simulink model "SF052A_SnsrOffsCorrn"  (R2013b)
settings: Solver=FixedStepDiscrete  SolverMode=SingleTasking  StartTime=0.0  StopTime=1  FixedStep=0.002  RelTol=1e-3
undefined symbols (not defined in the file): SnsrOffsCorrnHwAgLrndOffsLim, SnsrOffsCorrnHwTqLrndOffsLim, SnsrOffsCorrnOffsEna, SnsrOffsCorrnVehYawRateLrndOffsLim
libraries: NxtrLim x6, simulink x2
settings Model: Creator=SumitG  LastModifiedBy=TZ5743
settings SolverCC: AutoInsertRateTranBlk=on  InsertRTBMode=Always
settings DataIOCC: LimitDataPoints=off  SaveFormat=Structure  ReturnWorkspaceOutputs=on
settings OptimizationCC: BlockReduction=off  InlineParams=on  ZeroExternalMemoryAtStartup=off  ZeroInternalMemoryAtStartup=off  OptimizeModelRefInitCode=on  LifeSpan=1
settings DebuggingCC: SignalInfNanChecking=error  SignalRangeChecking=warning  UnderspecifiedInitializationDetection=Simplified  SolverPrmCheckMsg=error  InheritedTsInSrcMsg=error  DiscreteInheritContinuousMsg=error  SingleTaskRateTransMsg=error  TasksWithSamePriorityMsg=error  SigSpecEnsureSampleTimeMsg=error  CheckMatrixSingularityMsg=error  ParameterUnderflowMsg=error  ParameterPrecisionLossMsg=error  ParameterTunabilityLossMsg=error  FixptConstUnderflowMsg=warning  FixptConstOverflowMsg=warning  VectorMatrixConversionMsg=error  SignalLabelMismatchMsg=error  UnconnectedInputMsg=error  UnconnectedOutputMsg=error  UnconnectedLineMsg=error  SFcnCompatibilityMsg=error  UniqueDataStoreMsg=warning  BusObjectLabelMismatch=error  RootOutportRequireBusObject=error  AssertControl=DisableAll  ModelReferenceIOMsg=error  ModelReferenceVersionMismatchMessage=warning  ModelReferenceIOMismatchMessage=error  ModelReferenceCSMismatchMessage=warning  ModelReferenceDataLoggingMessage=error  StateNameClashWarn=warning  StrictBusMsg=ErrorOnBusTreatedAsVector  NonBusSignalsTreatedAsBus=error  SFUnexpectedBacktrackingDiag=error  SFInvalidInputDataAccessInChartInitDiag=error  SFNoUnconditionalDefaultTransitionDiag=error  SFTransitionOutsideNaturalParentDiag=error  SFUnconditionalTransitionShadowingDiag=error  SFUndirectedBroadcastEventsDiag=error
settings ModelReferenceCC: ModelReferenceNumInstancesAllowed=Single
settings RTWCC: SystemTargetFile=autosar.tlc  GenCodeOnly=on  TemplateMakefile=ert_default_tmf  Description=AUTOSAR  GenerateReport=on  ProcessScript=autosar_make_rtw_hook  LaunchReport=on
settings CodeAppCC: GenerateComments=off  IgnoreCustomStorageClasses=off  CustomSymbolStrType=$N$R$M  CustomSymbolStrBlkIO=$N$M  SimulinkBlockComments=off
settings STFCustomTargetCC: ParMdlRefBuildCompliant=on  CompOptLevelCompliant=on  IncludeMdlTerminateFcn=off  CombineOutputUpdateFcns=on  SuppressErrorStatus=on  ERTFirstTimeCompliant=on  ERTCustomFileBanners=on  SupportNonFinite=off  SupportComplex=off  SupportContinuousTime=off  SupportNonInlinedSFcns=off  MATLABClassNameForMDSCustomization=Simulink.SoftwareTarget.ERTCustomization  AutosarCompliant=on  GRTInterface=off  SystemTargetFile=autosar.tlc
settings ERTTargetCC: CodeReplacementLibrary=ANSI_C  ConcurrentExecutionCompliant=off  IncludeMdlTerminateFcn=off  SuppressErrorStatus=on  SupportNonFinite=off  SupportComplex=off  ModelStepFunctionPrototypeControlCompliant=off  CPPClassGenCompliant=off  AutosarCompliant=on  InlinedParameterPlacement=NonHierarchical  ERTCustomFileTemplate=example_file_process.tlc  EnableUserReplacementTypes=on

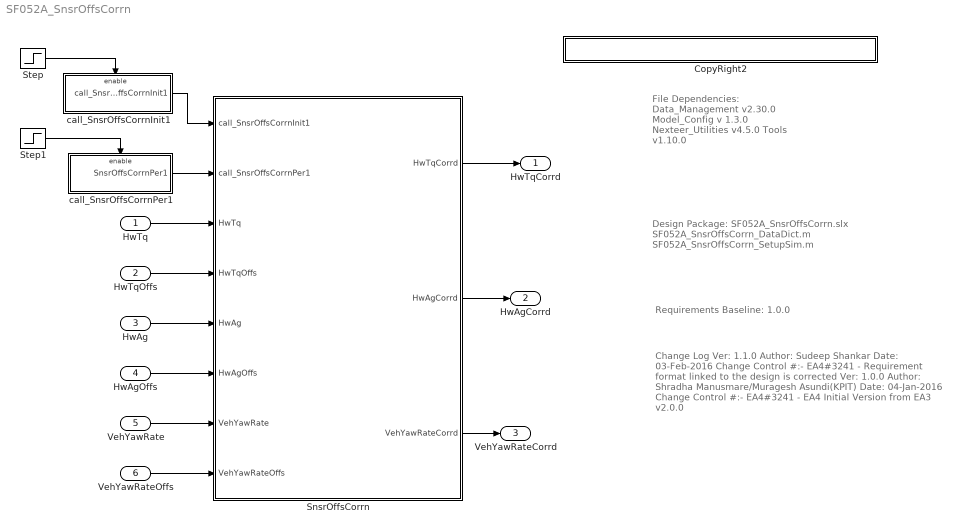
== system SF052A_SnsrOffsCorrn ==
  note: File Dependencies:
      |
      | Data_Management v2.30.0
      | Model_Config v 1.3.0
      | Nexteer_Utilities v4.5.0
      | Tools v1.10.0
  note: Requirements Baseline: 1.0.0
  note: Design Package:
      | SF052A_SnsrOffsCorrn.slx
      | SF052A_SnsrOffsCorrn_DataDict.m
      | SF052A_SnsrOffsCorrn_SetupSim.m
  note: Change Log
      |
      | Ver: 1.1.0
      | Author: Sudeep Shankar
      | Date: 03-Feb-2016
      | Change Control #:- EA4#3241
      | - Requirement format linked to the design is corrected
      |
      | Ver: 1.0.0
      | Author: Shradha Manusmare/Muragesh Asundi(KPIT)
      | Date: 04-Jan-2016
      | Change Control #:- EA4#3241
      | - EA4 Initial Version from EA3 v2.0.0
  HwTq : Inport  RequirementInfo={} %GIDa_2cd6e272_0df7_4175_9761_7c22e4c47b1c
  HwTqOffs : Inport  RequirementInfo={} %GIDa_54a2ce7e_9bb3_43b4_b9bf_3347b6fc5bcb  Port=2
  HwAg : Inport  RequirementInfo={} %GIDa_eed449fb_96e4_4476_834f_f50e1c62bf51  Port=3
  HwAgOffs : Inport  RequirementInfo={} %GIDa_50720404_89e5_4c59_9f63_6b50f8eae543  Port=4
  VehYawRate : Inport  RequirementInfo={} %GIDa_c6d0fb8d_2bf0_45a9_af32_27cacd4678ab  Port=5
  VehYawRateOffs : Inport  RequirementInfo={} %GIDa_e4fac660_fc81_4d67_abb0_5d2918f20bf2  Port=6
  CopyRight2 : Subsystem  Description=|  mask(Copyright Information){none=on}
      | Copyright info block.                                               
      |                                                                     
      | Place copyright information at the top of every subsystem in design.
      mask prompts: none "No parameters"
      mask help: Place copyright information at the top of every subsystem in design.
      mask Display:
      | NxtrConf = 'Nexteer Confidential';
      | 
      | sys = bdroot; %handle for the current model ("system")
      | first = get_param(sys,'Created');
      | first = first(end-3:end);  %year is last four digits
      | 
      | last = get_param(sys,'LastModifiedDate');
      | if isempty(last)
      |     last = datestr(now,'yyyy');
      | else
      |     last = last(end-3:end);
      | end
      | 
      | if strcmp(first,last)
      |     fprintf('%s -- Copyright %s Nexteer',NxtrConf,first)
      | else
      |     fprintf('%s -- %s%s- %s Nexteer',NxtrConf,char(169),first,last)
      | end
  SnsrOffsCorrn : Subsystem  RequirementInfo="{'linktype_rmi_doors' '0000bab4 (/E-STEER Core/SubSystem Specifications/Application Functions/SF052A Sensor Offset Correction  v0p2 150831)' '#SF052A_10' 'true' 'REQ:  SF052A_10' '' } %GIDa_ea5d6bfe_7895_439c_b9de_069ac848c9e6"
  Step : Step  Before=1  After=0  SampleTime=0
  Step1 : Step  SampleTime=0
  call_SnsrOffsCorrnInit1 : Subsystem  TreatAsAtomicUnit=on
  call_SnsrOffsCorrnPer1 : Subsystem  TreatAsAtomicUnit=on
  HwTqCorrd : Outport
  HwAgCorrd : Outport  Port=2
  VehYawRateCorrd : Outport  Port=3
  wires:
  SnsrOffsCorrn/3(VehYawRateCorrd) -> VehYawRateCorrd/1
  SnsrOffsCorrn/2(HwAgCorrd) -> HwAgCorrd/1
  SnsrOffsCorrn/1(HwTqCorrd) -> HwTqCorrd/1
  call_SnsrOffsCorrnInit1/1(call_SnsrOffsCorrnInit1) -> SnsrOffsCorrn/1(call_SnsrOffsCorrnInit1)
  HwAgOffs/1 -> SnsrOffsCorrn/6(HwAgOffs)
  VehYawRateOffs/1 -> SnsrOffsCorrn/8(VehYawRateOffs)
  VehYawRate/1 -> SnsrOffsCorrn/7(VehYawRate)
  HwAg/1 -> SnsrOffsCorrn/5(HwAg)
  HwTqOffs/1 -> SnsrOffsCorrn/4(HwTqOffs)
  HwTq/1 -> SnsrOffsCorrn/3(HwTq)
  Step/1 -> call_SnsrOffsCorrnInit1/Enable
  call_SnsrOffsCorrnPer1/1(SnsrOffsCorrnPer1) -> SnsrOffsCorrn/2(call_SnsrOffsCorrnPer1)
  Step1/1 -> call_SnsrOffsCorrnPer1/Enable

== system SF052A_SnsrOffsCorrn/CopyRight2 ==

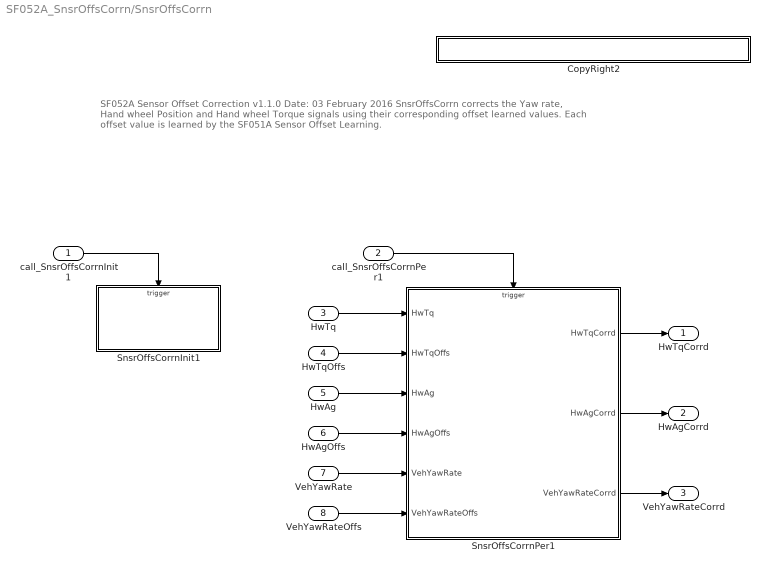
== system SF052A_SnsrOffsCorrn/SnsrOffsCorrn ==
  note: SF052A  Sensor Offset Correction
      | v1.1.0 								                                                                     Date: 03 February 2016
      |
      | SnsrOffsCorrn corrects the Yaw rate, Hand wheel Position and Hand wheel Torque signals using their
      | corresponding offset learned values. Each offset value is learned by the SF051A Sensor Offset Learning.
  call_SnsrOffsCorrnInit1 : Inport
  call_SnsrOffsCorrnPer1 : Inport  RequirementInfo="{'linktype_rmi_doors' '0000bab4 (/E-STEER Core/SubSystem Specifications/Application Functions/SF052A Sensor Offset Correction  v0p2 150831)' '#SF052A_56' 'true' 'REQ:  SF052A_56' '' } %GIDa_c7ebcd4c_7a0e_430e_914f_69a33bdc4f8e"  Port=2
  HwTq : Inport  RequirementInfo="{'linktype_rmi_doors' '0000bab4 (/E-STEER Core/SubSystem Specifications/Application Functions/SF052A Sensor Offset Correction  v0p2 150831)' '#SF052A_10' 'true' 'REQ:  SF052A_10' '' } %GIDa_886c7520_3b64_4a4e_b91f_bd52fc6cdafc"  Port=3
  HwTqOffs : Inport  RequirementInfo="{'linktype_rmi_doors' '0000bab4 (/E-STEER Core/SubSystem Specifications/Application Functions/SF052A Sensor Offset Correction  v0p2 150831)' '#SF052A_13' 'true' 'REQ:  SF052A_13' '' } %GIDa_0789263f_55f5_4e30_882e_ed1743b93406"  Port=4
  HwAg : Inport  RequirementInfo="{'linktype_rmi_doors' '0000bab4 (/E-STEER Core/SubSystem Specifications/Application Functions/SF052A Sensor Offset Correction  v0p2 150831)' '#SF052A_11' 'true' 'REQ:  SF052A_11' '' } %GIDa_98e8cd6b_ab1c_44ad_b544_e07a839ca543"  Port=5
  HwAgOffs : Inport  RequirementInfo="{'linktype_rmi_doors' '0000bab4 (/E-STEER Core/SubSystem Specifications/Application Functions/SF052A Sensor Offset Correction  v0p2 150831)' '#SF052A_14' 'true' 'REQ:  SF052A_14' '' } %GIDa_35d31cf1_93f6_46eb_aefe_bfa7895b93aa"  Port=6
  VehYawRate : Inport  RequirementInfo="{'linktype_rmi_doors' '0000bab4 (/E-STEER Core/SubSystem Specifications/Application Functions/SF052A Sensor Offset Correction  v0p2 150831)' '#SF052A_12' 'true' 'REQ:  SF052A_12' '' } %GIDa_f163533a_1fd4_4cf7_966b_304b3abdf020"  Port=7
  VehYawRateOffs : Inport  RequirementInfo="{'linktype_rmi_doors' '0000bab4 (/E-STEER Core/SubSystem Specifications/Application Functions/SF052A Sensor Offset Correction  v0p2 150831)' '#SF052A_15' 'true' 'REQ:  SF052A_15' '' } %GIDa_349c3e39_d0d8_4839_8edd_a04b0f97528a"  Port=8
  CopyRight2 : Subsystem  Description=|  mask(Copyright Information){none=on}
      | Copyright info block.                                               
      |                                                                     
      | Place copyright information at the top of every subsystem in design.
      mask prompts: none "No parameters"
      mask help: Place copyright information at the top of every subsystem in design.
      mask Display:
      | NxtrConf = 'Nexteer Confidential';
      | 
      | sys = bdroot; %handle for the current model ("system")
      | first = get_param(sys,'Created');
      | first = first(end-3:end);  %year is last four digits
      | 
      | last = get_param(sys,'LastModifiedDate');
      | if isempty(last)
      |     last = datestr(now,'yyyy');
      | else
      |     last = last(end-3:end);
      | end
      | 
      | if strcmp(first,last)
      |     fprintf('%s -- Copyright %s Nexteer',NxtrConf,first)
      | else
      |     fprintf('%s -- %s%s- %s Nexteer',NxtrConf,char(169),first,last)
      | end
  SnsrOffsCorrnInit1 : Subsystem  TreatAsAtomicUnit=on
  SnsrOffsCorrnPer1 : Subsystem  TreatAsAtomicUnit=on
  HwTqCorrd : Outport  RequirementInfo="{'linktype_rmi_doors' '0000bab4 (/E-STEER Core/SubSystem Specifications/Application Functions/SF052A Sensor Offset Correction  v0p2 150831)' '#SF052A_17' 'true' 'REQ:  SF052A_17' '' } %GIDa_182c97d9_5f7d_4d89_81b8_b7d4c7ce856d"
  HwAgCorrd : Outport  RequirementInfo="{'linktype_rmi_doors' '0000bab4 (/E-STEER Core/SubSystem Specifications/Application Functions/SF052A Sensor Offset Correction  v0p2 150831)' '#SF052A_18' 'true' 'REQ:  SF052A_18' '' } %GIDa_122c88ba_5244_46f5_838e_7cffdb4a64bf"  Port=2
  VehYawRateCorrd : Outport  RequirementInfo="{'linktype_rmi_doors' '0000bab4 (/E-STEER Core/SubSystem Specifications/Application Functions/SF052A Sensor Offset Correction  v0p2 150831)' '#SF052A_19' 'true' 'REQ:  SF052A_19' '' } %GIDa_98fd8efd_54d6_4bd4_9a2d_dfa8e7aa3144"  Port=3
  wires:
  call_SnsrOffsCorrnPer1/1 -> SnsrOffsCorrnPer1/Trigger
  SnsrOffsCorrnPer1/1(HwTqCorrd) -> HwTqCorrd/1
  SnsrOffsCorrnPer1/2(HwAgCorrd) -> HwAgCorrd/1
  SnsrOffsCorrnPer1/3(VehYawRateCorrd) -> VehYawRateCorrd/1
  VehYawRateOffs/1 -> SnsrOffsCorrnPer1/6(VehYawRateOffs)
  VehYawRate/1 -> SnsrOffsCorrnPer1/5(VehYawRate)
  HwAgOffs/1 -> SnsrOffsCorrnPer1/4(HwAgOffs)
  HwAg/1 -> SnsrOffsCorrnPer1/3(HwAg)
  HwTqOffs/1 -> SnsrOffsCorrnPer1/2(HwTqOffs)
  HwTq/1 -> SnsrOffsCorrnPer1/1(HwTq)
  call_SnsrOffsCorrnInit1/1 -> SnsrOffsCorrnInit1/Trigger

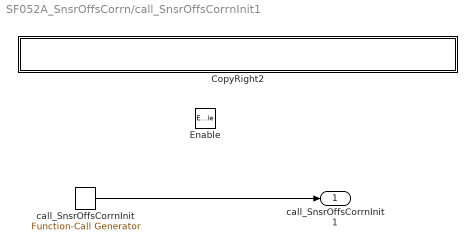
== system SF052A_SnsrOffsCorrn/call_SnsrOffsCorrnInit1 ==
  Enable : EnablePort
  CopyRight2 : Subsystem  Description=|  mask(Copyright Information){none=on}
      | Copyright info block.                                               
      |                                                                     
      | Place copyright information at the top of every subsystem in design.
      mask prompts: none "No parameters"
      mask help: Place copyright information at the top of every subsystem in design.
      mask Display:
      | NxtrConf = 'Nexteer Confidential';
      | 
      | sys = bdroot; %handle for the current model ("system")
      | first = get_param(sys,'Created');
      | first = first(end-3:end);  %year is last four digits
      | 
      | last = get_param(sys,'LastModifiedDate');
      | if isempty(last)
      |     last = datestr(now,'yyyy');
      | else
      |     last = last(end-3:end);
      | end
      | 
      | if strcmp(first,last)
      |     fprintf('%s -- Copyright %s Nexteer',NxtrConf,first)
      | else
      |     fprintf('%s -- %s%s- %s Nexteer',NxtrConf,char(169),first,last)
      | end
  "call_SnsrOffsCorrnInit " : simulink/Ports & Subsystems/Function-Call Generator  sample_time=0  numberOfIterations=1
  call_SnsrOffsCorrnInit1 : Outport
  wires:
  "call_SnsrOffsCorrnInit "/1 -> call_SnsrOffsCorrnInit1/1

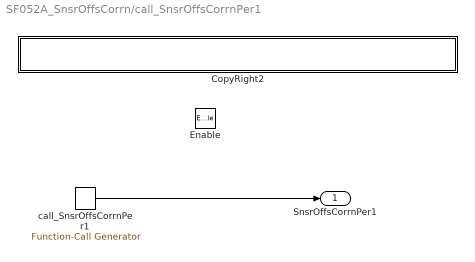
== system SF052A_SnsrOffsCorrn/call_SnsrOffsCorrnPer1 ==
  Enable : EnablePort
  CopyRight2 : Subsystem  Description=|  mask(Copyright Information){none=on}
      | Copyright info block.                                               
      |                                                                     
      | Place copyright information at the top of every subsystem in design.
      mask prompts: none "No parameters"
      mask help: Place copyright information at the top of every subsystem in design.
      mask Display:
      | NxtrConf = 'Nexteer Confidential';
      | 
      | sys = bdroot; %handle for the current model ("system")
      | first = get_param(sys,'Created');
      | first = first(end-3:end);  %year is last four digits
      | 
      | last = get_param(sys,'LastModifiedDate');
      | if isempty(last)
      |     last = datestr(now,'yyyy');
      | else
      |     last = last(end-3:end);
      | end
      | 
      | if strcmp(first,last)
      |     fprintf('%s -- Copyright %s Nexteer',NxtrConf,first)
      | else
      |     fprintf('%s -- %s%s- %s Nexteer',NxtrConf,char(169),first,last)
      | end
  "call_SnsrOffsCorrnPer1 " : simulink/Ports & Subsystems/Function-Call Generator  sample_time=0  numberOfIterations=1
  SnsrOffsCorrnPer1 : Outport
  wires:
  "call_SnsrOffsCorrnPer1 "/1 -> SnsrOffsCorrnPer1/1

== system SF052A_SnsrOffsCorrn/SnsrOffsCorrn/CopyRight2 ==

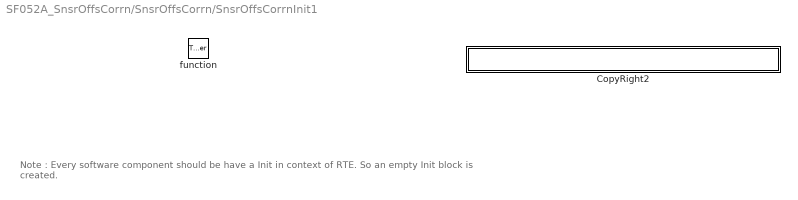
== system SF052A_SnsrOffsCorrn/SnsrOffsCorrn/SnsrOffsCorrnInit1 ==
  note: Note : Every software component should be have a Init in context of RTE. So an empty Init block is created.
  function : TriggerPort  TriggerType=function-call
  CopyRight2 : Subsystem  Description=|  mask(Copyright Information){none=on}
      | Copyright info block.                                               
      |                                                                     
      | Place copyright information at the top of every subsystem in design.
      mask prompts: none "No parameters"
      mask help: Place copyright information at the top of every subsystem in design.
      mask Display:
      | NxtrConf = 'Nexteer Confidential';
      | 
      | sys = bdroot; %handle for the current model ("system")
      | first = get_param(sys,'Created');
      | first = first(end-3:end);  %year is last four digits
      | 
      | last = get_param(sys,'LastModifiedDate');
      | if isempty(last)
      |     last = datestr(now,'yyyy');
      | else
      |     last = last(end-3:end);
      | end
      | 
      | if strcmp(first,last)
      |     fprintf('%s -- Copyright %s Nexteer',NxtrConf,first)
      | else
      |     fprintf('%s -- %s%s- %s Nexteer',NxtrConf,char(169),first,last)
      | end

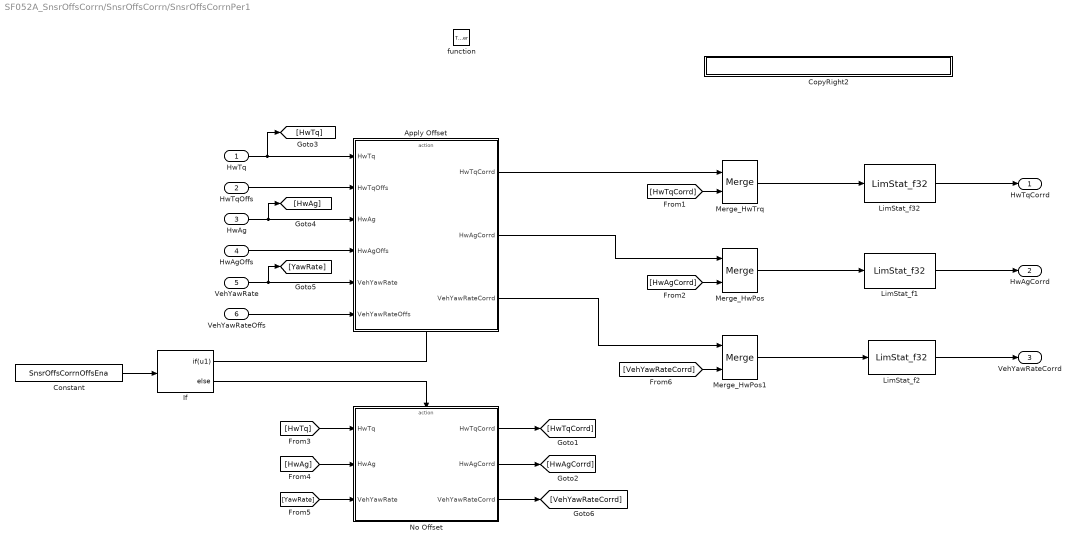
== system SF052A_SnsrOffsCorrn/SnsrOffsCorrn/SnsrOffsCorrnPer1 ==
  HwTq : Inport
  HwTqOffs : Inport  Port=2
  HwAg : Inport  Port=3
  HwAgOffs : Inport  Port=4
  VehYawRate : Inport  Port=5
  VehYawRateOffs : Inport  Port=6
  function : TriggerPort  TriggerType=function-call
  Apply Offset : Subsystem  TreatAsAtomicUnit=on
  Constant : Constant  RequirementInfo="{'linktype_rmi_doors' '0000bab4 (/E-STEER Core/SubSystem Specifications/Application Functions/SF052A Sensor Offset Correction  v0p2 150831)' '#SF052A_59' 'true' 'REQ:  SF052A_59' '' } %GIDa_2ea6c251_add8_4fde_8222_930c6875a31a"  Value=SnsrOffsCorrnOffsEna  OutDataTypeStr=boolean
  CopyRight2 : Subsystem  Description=|  mask(Copyright Information){none=on}
      | Copyright info block.                                               
      |                                                                     
      | Place copyright information at the top of every subsystem in design.
      mask prompts: none "No parameters"
      mask help: Place copyright information at the top of every subsystem in design.
      mask Display:
      | NxtrConf = 'Nexteer Confidential';
      | 
      | sys = bdroot; %handle for the current model ("system")
      | first = get_param(sys,'Created');
      | first = first(end-3:end);  %year is last four digits
      | 
      | last = get_param(sys,'LastModifiedDate');
      | if isempty(last)
      |     last = datestr(now,'yyyy');
      | else
      |     last = last(end-3:end);
      | end
      | 
      | if strcmp(first,last)
      |     fprintf('%s -- Copyright %s Nexteer',NxtrConf,first)
      | else
      |     fprintf('%s -- %s%s- %s Nexteer',NxtrConf,char(169),first,last)
      | end
  If : If  RequirementInfo="{'linktype_rmi_doors' '0000bab4 (/E-STEER Core/SubSystem Specifications/Application Functions/SF052A Sensor Offset Correction  v0p2 150831)' '#SF052A_59' 'true' 'REQ:  SF052A_59' '' } %GIDa_2324c2e3_bcd9_4140_a9db_9a8142331170"  IfExpression=u1
  LimStat_f1 : NxtrLim/LimStat_f32  RequirementInfo="{'linktype_rmi_doors' '0000bab4 (/E-STEER Core/SubSystem Specifications/Application Functions/SF052A Sensor Offset Correction  v0p2 150831)' '#SF052A_36' 'true' 'REQ:  SF052A_36' '' } %GIDa_c146a09b_42a0_4475_9c71_a8af706049e4"  LoLim=HWAGLOLIM_HWDEG_F32  HiLim=HWAGHILIM_HWDEG_F32
      settings: AttributesFormatString=|
      | Low Limit: %<LoLim>
      | High Limit:%<HiLim>
  LimStat_f2 : NxtrLim/LimStat_f32  RequirementInfo="{'linktype_rmi_doors' '0000bab4 (/E-STEER Core/SubSystem Specifications/Application Functions/SF052A Sensor Offset Correction  v0p2 150831)' '#SF052A_37' 'true' 'REQ:  SF052A_37' '' } %GIDa_c30e3b2b_2f7c_4b91_b252_a338ad55317b"  LoLim=VEHYAWRATELOLIM_VEHDEGPERSEC_F32  HiLim=VEHYAWRATEHILIM_VEHDEGPERSEC_F32
      settings: AttributesFormatString=|
      | Low Limit: %<LoLim>
      | High Limit:%<HiLim>
  LimStat_f32 : NxtrLim/LimStat_f32  RequirementInfo="{'linktype_rmi_doors' '0000bab4 (/E-STEER Core/SubSystem Specifications/Application Functions/SF052A Sensor Offset Correction  v0p2 150831)' '#SF052A_35' 'true' 'REQ:  SF052A_35' '' } %GIDa_66be3942_6c95_4b2c_b34d_b042724e9ab2"  LoLim=ELECGLBPRM_HWTQSATNLOWRLIM_HWNWTMTR_F32  HiLim=ELECGLBPRM_HWTQSATNUPPRLIM_HWNWTMTR_F32
      settings: AttributesFormatString=|
      | Low Limit: %<LoLim>
      | High Limit:%<HiLim>
  Merge_HwPos : Merge
  Merge_HwPos1 : Merge
  Merge_HwTrq : Merge
  No Offset : Subsystem  TreatAsAtomicUnit=on
  HwTqCorrd : Outport
  HwAgCorrd : Outport  Port=2
  VehYawRateCorrd : Outport  Port=3
  wires:
  Constant/1 -> If/1
  Merge_HwTrq/1 -> LimStat_f32/1
  LimStat_f32/1 -> HwTqCorrd/1
  Merge_HwPos/1 -> LimStat_f1/1
  LimStat_f1/1 -> HwAgCorrd/1
  Merge_HwPos1/1 -> LimStat_f2/1
  LimStat_f2/1 -> VehYawRateCorrd/1
  HwTq/1 -> [HwTq], Apply Offset/1(HwTq)
  HwTqOffs/1 -> Apply Offset/2(HwTqOffs)
  HwAg/1 -> Apply Offset/3(HwAg), [HwAg]
  HwAgOffs/1 -> Apply Offset/4(HwAgOffs)
  VehYawRate/1 -> [YawRate], Apply Offset/5(VehYawRate)
  VehYawRateOffs/1 -> Apply Offset/6(VehYawRateOffs)
  If/1 -> Apply Offset/Action
  [HwTq] -> No Offset/1(HwTq)
  [HwAg] -> No Offset/2(HwAg)
  [YawRate] -> No Offset/3(VehYawRate)
  If/2 -> No Offset/Action
  Apply Offset/1(HwTqCorrd) -> Merge_HwTrq/1
  Apply Offset/2(HwAgCorrd) -> Merge_HwPos/1
  Apply Offset/3(VehYawRateCorrd) -> Merge_HwPos1/1
  No Offset/1(HwTqCorrd) -> [HwTqCorrd]
  No Offset/2(HwAgCorrd) -> [HwAgCorrd]
  No Offset/3(VehYawRateCorrd) -> [VehYawRateCorrd]
  [HwTqCorrd] -> Merge_HwTrq/2
  [HwAgCorrd] -> Merge_HwPos/2
  [VehYawRateCorrd] -> Merge_HwPos1/2

== system SF052A_SnsrOffsCorrn/call_SnsrOffsCorrnInit1/CopyRight2 ==

== system SF052A_SnsrOffsCorrn/call_SnsrOffsCorrnPer1/CopyRight2 ==

== system SF052A_SnsrOffsCorrn/SnsrOffsCorrn/SnsrOffsCorrnInit1/CopyRight2 ==

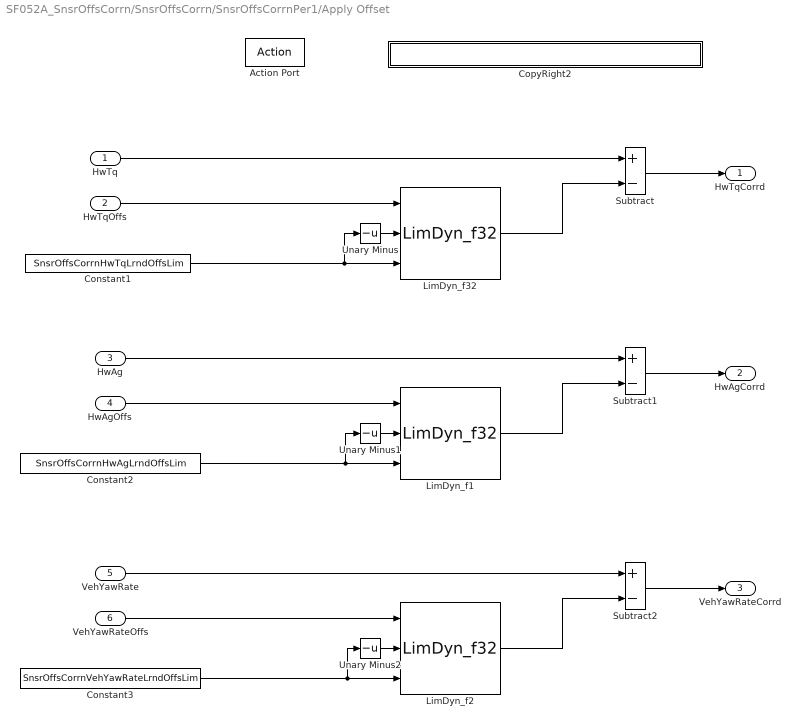
== system SF052A_SnsrOffsCorrn/SnsrOffsCorrn/SnsrOffsCorrnPer1/Apply Offset ==
  HwTq : Inport
  HwTqOffs : Inport  RequirementInfo={} %GIDa_208833cf_6878_470b_b6db_b869c72ce382  Port=2
  HwAg : Inport  Port=3
  HwAgOffs : Inport  RequirementInfo={} %GIDa_13fd176b_bd90_4d1e_898c_b4cb84dd90d3  Port=4
  VehYawRate : Inport  Port=5
  VehYawRateOffs : Inport  RequirementInfo={} %GIDa_c6aad98d_57dc_4e55_93b2_43b7f5e68072  Port=6
  Action Port : ActionPort  ActionType=then
  Constant1 : Constant  RequirementInfo="{'linktype_rmi_doors' '0000bab4 (/E-STEER Core/SubSystem Specifications/Application Functions/SF052A Sensor Offset Correction  v0p2 150831)' '#SF052A_28' 'true' 'REQ:  SF052A_28' '' ; 'linktype_rmi_doors' '0000bab4 (/E-STEER Core/SubSystem Specifications/Application Functions/SF052A Sensor Offset Correction  v0p2 150831)' '#SF052A_59' 'true' 'REQ:  SF052A_59' '' } %GIDa_c02cbdf8_d780_4ec2_988f_a7f581d45f4e"  Value=SnsrOffsCorrnHwTqLrndOffsLim  OutDataTypeStr=single
  Constant2 : Constant  RequirementInfo="{'linktype_rmi_doors' '0000bab4 (/E-STEER Core/SubSystem Specifications/Application Functions/SF052A Sensor Offset Correction  v0p2 150831)' '#SF052A_29' 'true' 'REQ:  SF052A_29' '' ; 'linktype_rmi_doors' '0000bab4 (/E-STEER Core/SubSystem Specifications/Application Functions/SF052A Sensor Offset Correction  v0p2 150831)' '#SF052A_59' 'true' 'REQ:  SF052A_59' '' } %GIDa_84e76d09_10c3_4f45_963b_f70ffbb4b24a"  Value=SnsrOffsCorrnHwAgLrndOffsLim  OutDataTypeStr=single
  Constant3 : Constant  RequirementInfo="{'linktype_rmi_doors' '0000bab4 (/E-STEER Core/SubSystem Specifications/Application Functions/SF052A Sensor Offset Correction  v0p2 150831)' '#SF052A_30' 'true' 'REQ:  SF052A_30' '' ; 'linktype_rmi_doors' '0000bab4 (/E-STEER Core/SubSystem Specifications/Application Functions/SF052A Sensor Offset Correction  v0p2 150831)' '#SF052A_59' 'true' 'REQ:  SF052A_59' '' } %GIDa_e3eda51d_9ed4_441b_9c35_48416a4bd64d"  Value=SnsrOffsCorrnVehYawRateLrndOffsLim  OutDataTypeStr=single
  CopyRight2 : Subsystem  Description=|  mask(Copyright Information){none=on}
      | Copyright info block.                                               
      |                                                                     
      | Place copyright information at the top of every subsystem in design.
      mask prompts: none "No parameters"
      mask help: Place copyright information at the top of every subsystem in design.
      mask Display:
      | NxtrConf = 'Nexteer Confidential';
      | 
      | sys = bdroot; %handle for the current model ("system")
      | first = get_param(sys,'Created');
      | first = first(end-3:end);  %year is last four digits
      | 
      | last = get_param(sys,'LastModifiedDate');
      | if isempty(last)
      |     last = datestr(now,'yyyy');
      | else
      |     last = last(end-3:end);
      | end
      | 
      | if strcmp(first,last)
      |     fprintf('%s -- Copyright %s Nexteer',NxtrConf,first)
      | else
      |     fprintf('%s -- %s%s- %s Nexteer',NxtrConf,char(169),first,last)
      | end
  LimDyn_f1 : NxtrLim/LimDyn_f32
  LimDyn_f2 : NxtrLim/LimDyn_f32
  LimDyn_f32 : NxtrLim/LimDyn_f32
  Subtract : Sum  RequirementInfo="{'linktype_rmi_doors' '0000bab4 (/E-STEER Core/SubSystem Specifications/Application Functions/SF052A Sensor Offset Correction  v0p2 150831)' '#SF052A_31' 'true' 'REQ:  SF052A_31' '' } %GIDa_97e76b39_0074_4715_9b02_5b34293409b4"  Inputs=+-
  Subtract1 : Sum  RequirementInfo="{'linktype_rmi_doors' '0000bab4 (/E-STEER Core/SubSystem Specifications/Application Functions/SF052A Sensor Offset Correction  v0p2 150831)' '#SF052A_32' 'true' 'REQ:  SF052A_32' '' } %GIDa_29c43bfa_15d1_4944_b77e_3d3fcbed85e9"  Inputs=+-
  Subtract2 : Sum  RequirementInfo="{'linktype_rmi_doors' '0000bab4 (/E-STEER Core/SubSystem Specifications/Application Functions/SF052A Sensor Offset Correction  v0p2 150831)' '#SF052A_33' 'true' 'REQ:  SF052A_33' '' } %GIDa_4d734258_0917_4071_b468_5f3970d97b28"  Inputs=+-
  Unary Minus : UnaryMinus  RequirementInfo="{'linktype_rmi_doors' '0000bab4 (/E-STEER Core/SubSystem Specifications/Application Functions/SF052A Sensor Offset Correction  v0p2 150831)' '#SF052A_28' 'true' 'REQ:  SF052A_28' '' } %GIDa_9dad3694_480c_4199_8e32_179792dc55e6"
  Unary Minus1 : UnaryMinus  RequirementInfo="{'linktype_rmi_doors' '0000bab4 (/E-STEER Core/SubSystem Specifications/Application Functions/SF052A Sensor Offset Correction  v0p2 150831)' '#SF052A_29' 'true' 'REQ:  SF052A_29' '' } %GIDa_8e6f572f_425d_4f12_a1f7_6f6935bcde7d"
  Unary Minus2 : UnaryMinus  RequirementInfo="{'linktype_rmi_doors' '0000bab4 (/E-STEER Core/SubSystem Specifications/Application Functions/SF052A Sensor Offset Correction  v0p2 150831)' '#SF052A_30' 'true' 'REQ:  SF052A_30' '' } %GIDa_913df085_0e1b_4fac_9d50_f951467919cb"
  HwTqCorrd : Outport
  HwAgCorrd : Outport  Port=2
  VehYawRateCorrd : Outport  Port=3
  wires:
  HwTq/1 -> Subtract/1
  Constant1/1 -> Unary Minus/1, LimDyn_f32/3
  Unary Minus1/1 -> LimDyn_f1/2
  HwAg/1 -> Subtract1/1
  Constant2/1 -> Unary Minus1/1, LimDyn_f1/3
  VehYawRate/1 -> Subtract2/1
  Unary Minus/1 -> LimDyn_f32/2
  HwTqOffs/1 -> LimDyn_f32/1
  LimDyn_f32/1 -> Subtract/2
  HwAgOffs/1 -> LimDyn_f1/1
  LimDyn_f1/1 -> Subtract1/2
  VehYawRateOffs/1 -> LimDyn_f2/1
  Constant3/1 -> Unary Minus2/1, LimDyn_f2/3
  Unary Minus2/1 -> LimDyn_f2/2
  LimDyn_f2/1 -> Subtract2/2
  Subtract2/1 -> VehYawRateCorrd/1
  Subtract/1 -> HwTqCorrd/1
  Subtract1/1 -> HwAgCorrd/1

== system SF052A_SnsrOffsCorrn/SnsrOffsCorrn/SnsrOffsCorrnPer1/CopyRight2 ==

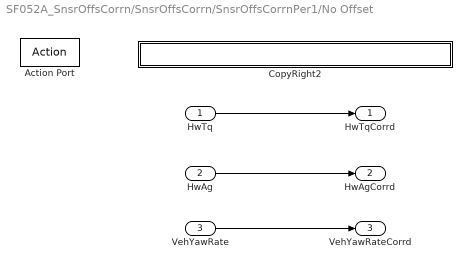
== system SF052A_SnsrOffsCorrn/SnsrOffsCorrn/SnsrOffsCorrnPer1/No Offset ==
  HwTq : Inport
  HwAg : Inport  Port=2
  VehYawRate : Inport  Port=3
  Action Port : ActionPort  ActionType=else
  CopyRight2 : Subsystem  Description=|  mask(Copyright Information){none=on}
      | Copyright info block.                                               
      |                                                                     
      | Place copyright information at the top of every subsystem in design.
      mask prompts: none "No parameters"
      mask help: Place copyright information at the top of every subsystem in design.
      mask Display:
      | NxtrConf = 'Nexteer Confidential';
      | 
      | sys = bdroot; %handle for the current model ("system")
      | first = get_param(sys,'Created');
      | first = first(end-3:end);  %year is last four digits
      | 
      | last = get_param(sys,'LastModifiedDate');
      | if isempty(last)
      |     last = datestr(now,'yyyy');
      | else
      |     last = last(end-3:end);
      | end
      | 
      | if strcmp(first,last)
      |     fprintf('%s -- Copyright %s Nexteer',NxtrConf,first)
      | else
      |     fprintf('%s -- %s%s- %s Nexteer',NxtrConf,char(169),first,last)
      | end
  HwTqCorrd : Outport
  HwAgCorrd : Outport  Port=2
  VehYawRateCorrd : Outport  Port=3
  wires:
  HwTq/1 -> HwTqCorrd/1
  HwAg/1 -> HwAgCorrd/1
  VehYawRate/1 -> VehYawRateCorrd/1

== system SF052A_SnsrOffsCorrn/SnsrOffsCorrn/SnsrOffsCorrnPer1/Apply Offset/CopyRight2 ==

== system SF052A_SnsrOffsCorrn/SnsrOffsCorrn/SnsrOffsCorrnPer1/No Offset/CopyRight2 ==
